simulink model "Microgrid_TLM_server"  (R2025b)
settings: Solver=FixedStepAuto  StartTime=0.0  StopTime=1  FixedStep=5e-7  RelTol=1e-3
InitFcn:
  | clear;
  | setup_two_pc_cosim();
  | clear Server_co Client_co
  | rehash;
  | release_two_pc_tcp_ports();
  | Zc = 45;
  | Vline = 380;%Rated RMS of Line Voltage
  | Vdc = 750;%DC voltage
  | Vac = sqrt(2)*Vline/sqrt(3);%Amplitude of Phase to Neutral Volatge
  | P = 10*10^(3);%Rate Power
  | f=50;%Rated Frequency
  | Wb=2*pi*f;%Rated Angular Frequency
  | fsw1=10e3;  %INV1 switching frequency
  | 
  | %Base Value of PU System
  | Vp=Vac;%Voltage
  | Ip=2/3*P/Vp;%Current
  | Zb = Vp/Ip;%Impedance
  | Lb=Zb/2/pi/f;%Inductance
  | Cb=1/(2*pi*f*Zb);%Capacitance
  | 
  | %Network Parameters
  | R1_pu=0.1/Zb;R1=R1_pu*Zb;
  | R2_pu=0.1/Zb;R2=R2_pu*Zb;
  | R3_pu=0.1/Zb;R3=R3_pu*Zb;
  | R4_pu=0.1/Zb;R4=R4_pu*Zb;
  | L1_pu=2e-3/Lb;L1=L1_pu*Lb;
  | L2_pu=2e-3/Lb;L2=L2_pu*Lb;
  | L3_pu=2e-3/Lb;L3=L3_pu*Lb;
  | L4_pu=2e-3/Lb;L4=L4_pu*Lb;
  | 
  | %Load Parameters
  | Rload1_pu=Vp/Ip/Zb;Rload1=Rload1_pu*Zb;
  | Rload2_pu=Vp/Ip/Zb;Rload2=Rload2_pu*Zb;
  | Rload3_pu=Vp/Ip/Zb;Rload3=Rload3_pu*Zb;
  | 
  | %Virtual Impedance
  | Rv_pu=0.05;
  | Xv_pu=0.2;
  | 
  | Lc=2.5e-3;
StopFcn:
  | %% StopFcn: save TLM server-side results
  | 
  | modelName = bdroot;
  | modelFile = get_param(modelName, 'FileName');
  | 
  | if isempty(modelFile)
  |     modelDir = pwd;
  | else
  |     modelDir = fileparts(modelFile);
  | end
  | 
  | resultDir = fullfile(modelDir, 'result');
  | 
  | if ~exist(resultDir, 'dir')
  |     mkdir(resultDir);
  | end
  | 
  | % Server-side workspace variables
  | variableNames = {
  |     'server_voltage'
  |     'server_current'
  |     'server_PQ'
  | };
  | 
  | serverTLMData = struct();
  | 
  | for k = 1:numel(variableNames)
  | 
  |     originalName = variableNames{k};
  |     saveName = [originalName, '_TLM'];
  | 
  |     if evalin('base', sprintf('exist(''%s'', ''var'')', originalName))
  |         serverTLMData.(saveName) = evalin('base', originalName);
  |     else
  |         warning( ...
  |             'StopFcn:MissingVariable', ...
  |             'Variable "%s" was not found in the base workspace.', ...
  |             originalName);
  |     end
  | end
  | 
  | % Save to result/server_TLM.mat
  | saveFile = fullfile(resultDir, 'server_TLM.mat');
  | save(saveFile, '-struct', 'serverTLMData');
  | 
  | fprintf('TLM server-side results saved to:\n%s\n', saveFile);
undefined symbols (not defined in the file or in its folder): DiscIntNeverNeededParam, Lline1
libraries: spsThreePhaseSeriesRLCBranchLib x14, spsControlledVoltageSourceLib x12, spsThreePhaseVIMeasurementLib x7, spsabctodq0Lib x6, slpidlib x4, spsThreePhaseBreakerLib x4, spsControlledCurrentSourceLib x3, SimplusGT x3, spsPower3phInstantaneousLib x2, spsdq0toabcLib x2, spsThreePhaseTransformerTwoWindingsLib x2, spsDistributedParametersLineLib x1
(part 1 of 2)
settings Model: Creator=L  LastModifiedBy=Zhai Xinjie
settings SolverCC: AlgebraicLoopSolver=TrustRegion
settings DataIOCC: LimitDataPoints=on  SaveFormat=Array  ReturnWorkspaceOutputs=off
settings OptimizationCC: ReuseModelBlockBuffer=off  LifeSpan=inf
settings DebuggingCC: UnderspecifiedInitializationDetection=Classic  MergeDetectMultiDrivingBlocksExec=none  SolverPrmCheckMsg=warning  UnconnectedInputMsg=warning  UnconnectedOutputMsg=warning  UnconnectedLineMsg=warning  StateNameClashWarn=warning  SFUnexpectedBacktrackingDiag=warning  SFNoUnconditionalDefaultTransitionDiag=warning  SFExecutionAtInitializationDiag=none  ArithmeticOperatorsInVariantConditions=warning
settings HardwareCC: ProdBitPerPointer=32.0  ProdBitPerSizeT=32.0  ProdBitPerPtrDiffT=32.0  ProdLargestAtomicFloat=None  ProdIntDivRoundTo=Undefined  ProdEndianess=Unspecified  ProdWordSize=32.0  ProdHWDeviceType=32-bit Generic
settings ModelReferenceCC: EnableRefExpFcnMdlSchedulingChecks=on  PropagateSignalLabelsOutOfModel=off
settings SFSimCC: SimUseLocalCustomCode=off  CustomCodeUndefinedFunction=UseInterfaceOnly
settings RTWCC: RTWUseLocalCustomCode=off  GPUComputeCapability=3.5  DLArmComputeVersion=19.05
settings CodeAppCC: StateflowObjectComments=on
settings GRTTargetCC: TargetLangStandard=C89/C90 (ANSI)
settings ConfigComp: CovMetricSettings=dw  CovSaveCumulativeToWorkspaceVar=on  CovSaveSingleToWorkspaceVar=on  CovExternalEMLEnable=off
settings SimscapeCC: SimscapeNormalizeSystem=off

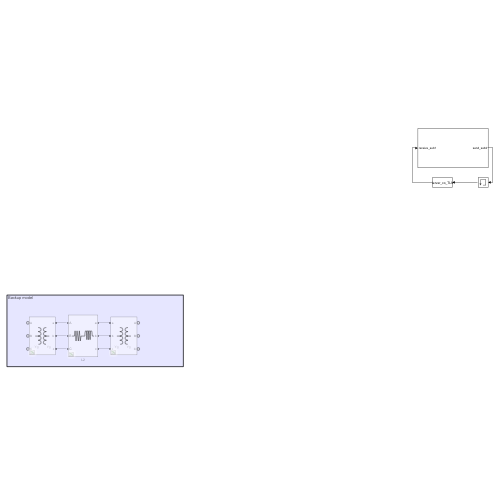
[thumbnail: Simulink's stored preview of the top-level diagram]
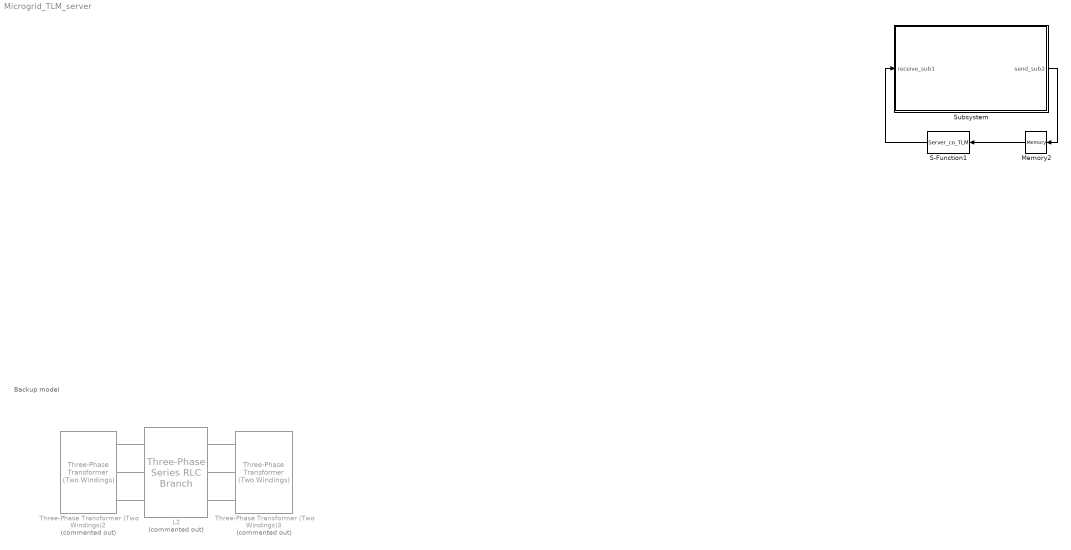
== system Microgrid_TLM_server ==
  note: Backup model
  L2 : spsThreePhaseSeriesRLCBranchLib/Three-Phase Series RLC Branch  Commented=on  LConnTagsString=A|B|C  RConnTagsString=A|B|C  BranchType=RL  Resistance=R2  Inductance=L2  Capacitance=1e-6  Measurements=None
  Memory2 : Memory
  S-Function1 : S-Function  FunctionName=Server_co_TLM  SFunctionDeploymentMode=off  EnableBusSupport=off
  Subsystem : Subsystem
  Three-Phase Transformer (Two Windings)2 : spsThreePhaseTransformerTwoWindingsLib/Three-Phase Transformer (Two Windings)  Commented=on  Winding1Connection=Yg  Winding2Connection=Yg  CoreType=Three single-phase transformers  SetSaturation=off  Hysteresis=off  DataFile='hysteresis'  SetInitialFlux=off  Measurements=None  UNITS=pu  NominalPower=[ 250e6 , 50 ]  Winding1=[ 380e3 , 0.002 , 0.08 ]  Winding2=[ 33e3 , 0.002 , 0.08 ]  Rm=500  Lm=500  L0=0.5  Saturation=[ 0,0 ; 0.0024,1.2 ; 1.0,1.52 ]  InitialFluxes=[ 0.8 , -0.8 , 0.7 ]  BreakLoop=off  DiscreteSolver=Trapezoidal iterative  DataType=off  TransfoNumber=1
  Three-Phase Transformer (Two Windings)3 : spsThreePhaseTransformerTwoWindingsLib/Three-Phase Transformer (Two Windings)  Commented=on  Winding1Connection=Yg  Winding2Connection=Yg  CoreType=Three single-phase transformers  SetSaturation=off  Hysteresis=off  DataFile='hysteresis'  SetInitialFlux=off  Measurements=None  UNITS=pu  NominalPower=[ 250e6 , 50 ]  Winding1=[ 33e3 , 0.002 , 0.08 ]  Winding2=[ 380 , 0.002 , 0.08 ]  Rm=500  Lm=500  L0=0.5  Saturation=[ 0,0 ; 0.0024,1.2 ; 1.0,1.52 ]  InitialFluxes=[ 0.8 , -0.8 , 0.7 ]  BreakLoop=off  DiscreteSolver=Trapezoidal iterative  DataType=off  TransfoNumber=1
  wires:
  Memory2/1 -> S-Function1/1
  Subsystem/1(send_sub2) -> Memory2/1
  S-Function1/1 -> Subsystem/1(receive_sub1)
  connections:
  Three-Phase Transformer (Two Windings)3/RConn1 -- L2/RConn1
  Three-Phase Transformer (Two Windings)3/RConn2 -- L2/RConn2
  Three-Phase Transformer (Two Windings)3/RConn3 -- L2/RConn3
  Three-Phase Transformer (Two Windings)2/RConn1 -- L2/LConn1
  Three-Phase Transformer (Two Windings)2/RConn2 -- L2/LConn2
  Three-Phase Transformer (Two Windings)2/RConn3 -- L2/LConn3

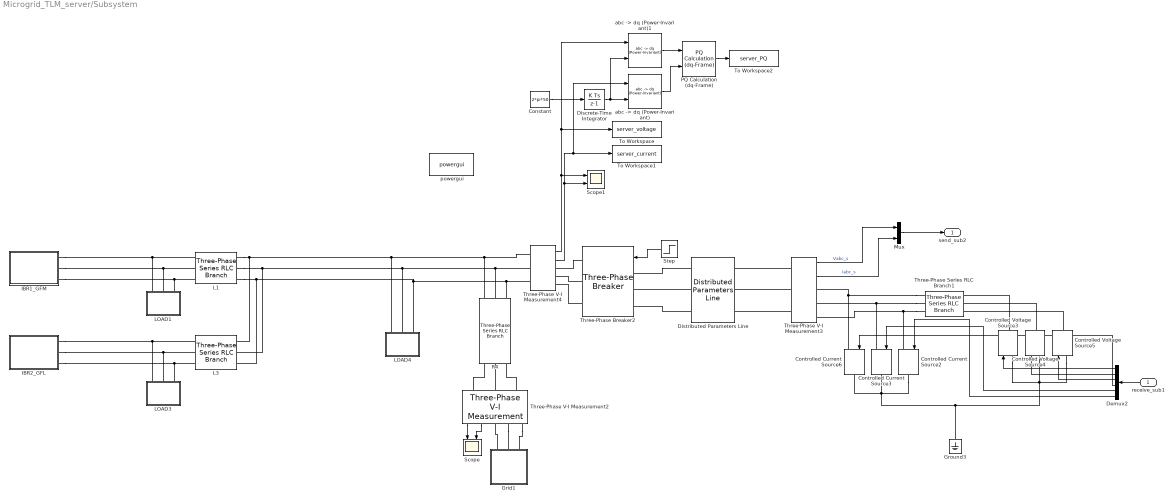
== system Microgrid_TLM_server/Subsystem ==
  receive_sub1 : Inport
  Constant : Constant  Value=2*pi*50
  Controlled Current Source2 : spsControlledCurrentSourceLib/Controlled Current Source  Initialize=on  Source_Type=AC  Amplitude=0  Phase=0  Frequency=0  Measurements=None
  Controlled Current Source3 : spsControlledCurrentSourceLib/Controlled Current Source  Initialize=on  Source_Type=AC  Amplitude=0  Phase=0  Frequency=0  Measurements=None
  Controlled Current Source6 : spsControlledCurrentSourceLib/Controlled Current Source  Initialize=on  Source_Type=AC  Amplitude=0  Phase=0  Frequency=0  Measurements=None
  Controlled Voltage Source3 : spsControlledVoltageSourceLib/Controlled Voltage Source  Initialize=on  Source_Type=AC  Amplitude=0  Phase=0  Frequency=0  Measurements=None
  Controlled Voltage Source4 : spsControlledVoltageSourceLib/Controlled Voltage Source  Initialize=on  Source_Type=AC  Amplitude=0  Phase=0  Frequency=0  Measurements=None
  Controlled Voltage Source5 : spsControlledVoltageSourceLib/Controlled Voltage Source  Initialize=on  Source_Type=AC  Amplitude=0  Phase=0  Frequency=0  Measurements=None
  Demux2 : Demux  Outputs=6
  Discrete-Time Integrator : DiscreteIntegrator  SampleTime=-1  ICPrevOutput=DiscIntNeverNeededParam  ICPrevScaledInput=DiscIntNeverNeededParam
  Distributed Parameters Line : spsDistributedParametersLineLib/Distributed Parameters Line  Phases=3  Length=0.3  Frequency=60  Resistance=[0.075 0.30]  Inductance=[0.30e-3 0.90e-3]  Capacitance=[148e-9 100e-9]  x1=[-3e-06 0 0 0;-2.5e-06 0 0 0;-2e-06 0 0 0;-1.5e-06 0 0 0;-1e-06 0 0 0;-5e-07 0 0 0]  x2=[-3e-06 0 0 0;-2.5e-06 0 0 0;-2e-06 0 0 0;-1.5e-06 0 0 0;-1e-06 0 0 0;-5e-07 0 0 0]  x3=[-3e-06 0 0 0;-2.5e-06 0 0 0;-2e-06 0 0 0;-1.5e-06 0 0 0;-1e-06 0 0 0;-5e-07 0 0 0]  x4=[-3e-06 0 0 0;-2.5e-06 0 0 0;-2e-06 0 0 0;-1.5e-06 0 0 0;-1e-06 0 0 0;-5e-07 0 0 0]  x5=2.84604989415154e-06  V1=ones(3,3)  V2=ones(3,3)  I1=ones(3,3)  I2=ones(3,3)  nHarmo=1  Measurements=None  Decoupling=off  VsMag0=0  VrMag0=0  VsAngle0=0  VrAngle0=0  IsMag0=0  IrMag0=0  IsAngle0=0  IrAngle0=0
      settings: LibrarySourceBlock=sps_lib/Power Grid Elements/Distributed Parameters Line
  Grid1 : Subsystem
  Ground3 : spsGroundLib/Ground  LConnTagsString=a
  IBR1_GFM : Subsystem
  IBR2_GFL : Subsystem
  L1 : spsThreePhaseSeriesRLCBranchLib/Three-Phase Series RLC Branch  LConnTagsString=A|B|C  RConnTagsString=A|B|C  BranchType=RL  Resistance=R1  Inductance=L1  Capacitance=1e-6  Measurements=None
  L3 : spsThreePhaseSeriesRLCBranchLib/Three-Phase Series RLC Branch  LConnTagsString=A|B|C  RConnTagsString=A|B|C  BranchType=RL  Resistance=R3  Inductance=L3  Capacitance=1e-6  Measurements=None
  LOAD1 : Subsystem
  LOAD3 : Subsystem
  LOAD4 : Subsystem
  Mux : Mux  Inputs=2
  PQ Calculation (dq-Frame) : SimplusGT/PQ Calculation (dq-Frame)  SystemSampleTime=-1  VariantActivationTime=update diagram  EmptyChoice=off  PassThrough=off  PassThroughVariantControl=(default)  EmptyChoiceVariantControl=(default)  AllowFlexibleInterface=on  Latency=0  AutoFrameSizeCalculation=off
      settings: SourceProductName=Simplus Grid Tool
  R4 : spsThreePhaseSeriesRLCBranchLib/Three-Phase Series RLC Branch  LConnTagsString=A|B|C  RConnTagsString=A|B|C  BranchType=RL  Resistance=R4  Inductance=L4  Capacitance=1e-6  Measurements=None
  Scope : Scope  NumInputPorts=2
      settings: ActiveDisplayYMinimum=-671.75144212722125  ActiveDisplayYMaximum=671.75144212722125
  Scope1 : Scope  NumInputPorts=2
      settings: ActiveDisplayYMinimum=-701.589020696881  ActiveDisplayYMaximum=701.610214034999  DataLoggingVariableName=ScopeData2
  Step : Step  Time=0.2  SampleTime=0
  Three-Phase Series RLC Branch1 : spsThreePhaseSeriesRLCBranchLib/Three-Phase Series RLC Branch  LConnTagsString=A|B|C  RConnTagsString=A|B|C  BranchType=R  Resistance=Zc  Inductance=1e-3  Capacitance=1e-6  Measurements=None
  Three-Phase V-I Measurement2 : spsThreePhaseVIMeasurementLib/Three-Phase V-I Measurement  VoltageMeasurement=phase-to-phase  SetLabelV=off  LabelV=Vabc1  Vpu=off  VpuLL=off  CurrentMeasurement=yes  SetLabelI=off  LabelI=Iabc3  Ipu=off  Pbase=100e6  Vbase=500e3  OutputType=Complex  PhasorSimulation=off  PSBequivalent=0
  Three-Phase V-I Measurement3 : spsThreePhaseVIMeasurementLib/Three-Phase V-I Measurement  VoltageMeasurement=phase-to-ground  SetLabelV=off  LabelV=Vabc_s  Vpu=off  VpuLL=off  CurrentMeasurement=yes  SetLabelI=off  LabelI=Iabc_s  Ipu=off  Pbase=100e6  Vbase=500e3  OutputType=Complex  PhasorSimulation=off  PSBequivalent=0
  Three-Phase V-I Measurement4 : spsThreePhaseVIMeasurementLib/Three-Phase V-I Measurement  VoltageMeasurement=phase-to-phase  SetLabelV=off  LabelV=Vabc1  Vpu=off  VpuLL=off  CurrentMeasurement=yes  SetLabelI=off  LabelI=Iabc3  Ipu=off  Pbase=100e6  Vbase=500e3  OutputType=Complex  PhasorSimulation=off  PSBequivalent=0
  Three-Phase Breaker2 : spsThreePhaseBreakerLib/Three-Phase Breaker  InitialState=open  SwitchA=on  SwitchB=on  SwitchC=on  SwitchTimes=1.5  External=on  BreakerResistance=0.01  SnubberResistance=1e6  SnubberCapacitance=inf  Measurements=None
  To Workspace : ToWorkspace  VariableName=server_voltage  SaveFormat=Timeseries  SampleTime=-1
  To Workspace1 : ToWorkspace  VariableName=server_current  SaveFormat=Timeseries  SampleTime=-1
  To Workspace2 : ToWorkspace  VariableName=server_PQ  SaveFormat=Timeseries  SampleTime=-1
  "abc -> dq (Power-Invariant)" : SimplusGT/abc -> dq (Power-Invariant)  SystemSampleTime=-1  VariantActivationTime=update diagram  EmptyChoice=off  PassThrough=off  PassThroughVariantControl=(default)  EmptyChoiceVariantControl=(default)  AllowFlexibleInterface=on  Latency=0  AutoFrameSizeCalculation=off
      settings: SourceProductName=Simplus Grid Tool
  "abc -> dq (Power-Invariant)1" : SimplusGT/abc -> dq (Power-Invariant)  SystemSampleTime=-1  VariantActivationTime=update diagram  EmptyChoice=off  PassThrough=off  PassThroughVariantControl=(default)  EmptyChoiceVariantControl=(default)  AllowFlexibleInterface=on  Latency=0  AutoFrameSizeCalculation=off
      settings: SourceProductName=Simplus Grid Tool
  powergui : spspowerguiLib/powergui  Priority=1  SimulationMode=Discrete  SampleTime=5e-7  frequency=60  Iterations=50  frequencyindice=0  Pbase=100e6  ErrMax=1e-4  UnitsV=kV  UnitsW=MW  buscounter=0  FunctionMessages=off  echomessages=off  EnableUseOfTLC=off  CurrentSourceSwitches=off  DisableSnubberDevices=off  DisableRonSwitches=off  DisableVfSwitches=off  DisplayEquations=off  AutomaticDiscreteSolvers=off  SolverType=Tustin/Backward Euler (TBE)  Interpol=off  ExternalGateDelay=off  methode=off  Ts=100  x0status=blocks  SPID=on  SwTol=0  HookPort=off  NonlinearTolerance=1e-4  nMaxIteration=100  ContinueOnMaxIteration=off  RestoreLinks=warning  ResistiveCurrentMeasurement=off  Frange=[0:2:500]  Ylog=off  Xlog=on  ShowGrid=off  save=off  variable=ZData  structure=0  ZoomFFT=off  StartTime=0.0  cycles=1  DisplayStyle=1  fundamental=60  FreqAxis=off  MaxFrequency=1000  frequencyindicesteady=1  RmsSteady=1  display=off
  send_sub2 : Outport
  wires:
  Three-Phase V-I Measurement2/2 -> Scope/2
  Three-Phase V-I Measurement2/1 -> Scope/1
  Step/1 -> Three-Phase Breaker2/1
  Demux2/3 -> Controlled Voltage Source5/1
  Demux2/4 -> Controlled Current Source6/1
  Demux2/2 -> Controlled Voltage Source4/1
  Three-Phase V-I Measurement3/2 -> Mux/2  "Iabc_s"
  Mux/1 -> send_sub2/1
  receive_sub1/1 -> Demux2/1
  Demux2/6 -> Controlled Current Source2/1
  Three-Phase V-I Measurement3/1 -> Mux/1  "Vabc_s"
  Demux2/1 -> Controlled Voltage Source3/1
  Demux2/5 -> Controlled Current Source3/1
  Three-Phase V-I Measurement4/1 -> Scope1/1, "abc -> dq (Power-Invariant)1"/1, To Workspace/1
  Three-Phase V-I Measurement4/2 -> Scope1/2, "abc -> dq (Power-Invariant)"/1, To Workspace1/1
  Discrete-Time Integrator/1 -> "abc -> dq (Power-Invariant)1"/2, "abc -> dq (Power-Invariant)"/2
  Constant/1 -> Discrete-Time Integrator/1
  "abc -> dq (Power-Invariant)1"/1 -> PQ Calculation (dq-Frame)/1
  "abc -> dq (Power-Invariant)"/1 -> PQ Calculation (dq-Frame)/2
  PQ Calculation (dq-Frame)/1 -> To Workspace2/1
  connections:
  IBR1_GFM/RConn2 -- L1/LConn2 -- LOAD1/LConn2
  Three-Phase V-I Measurement3/LConn1 -- Distributed Parameters Line/LConn1
  Grid1/LConn1 -- Three-Phase V-I Measurement2/RConn1
  LOAD4/LConn1 -- Three-Phase V-I Measurement4/LConn1 -- R4/LConn1 -- L1/RConn1 -- L3/RConn1
  Three-Phase V-I Measurement2/LConn3 -- R4/RConn3
  L1/LConn1 -- IBR1_GFM/RConn1 -- LOAD1/LConn1
  L1/RConn2 -- Three-Phase V-I Measurement4/LConn2 -- R4/LConn2 -- LOAD4/LConn2 -- L3/RConn2
  Distributed Parameters Line/RConn3 -- Three-Phase Breaker2/LConn3
  Three-Phase V-I Measurement2/RConn2 -- Grid1/LConn2
  IBR1_GFM/RConn3 -- L1/LConn3 -- LOAD1/LConn3
  L1/RConn3 -- L3/RConn3 -- LOAD4/LConn3 -- Three-Phase V-I Measurement4/LConn3 -- R4/LConn3
  Distributed Parameters Line/RConn1 -- Three-Phase Breaker2/LConn1
  LOAD3/LConn1 -- IBR2_GFL/RConn1 -- L3/LConn1
  IBR2_GFL/RConn2 -- LOAD3/LConn2 -- L3/LConn2
  Three-Phase V-I Measurement3/LConn2 -- Distributed Parameters Line/LConn2
  Distributed Parameters Line/RConn2 -- Three-Phase Breaker2/LConn2
  Three-Phase V-I Measurement3/LConn3 -- Distributed Parameters Line/LConn3
  Three-Phase V-I Measurement2/RConn3 -- Grid1/LConn3
  Three-Phase V-I Measurement2/LConn1 -- R4/RConn1
  IBR2_GFL/RConn3 -- LOAD3/LConn3 -- L3/LConn3
  Three-Phase V-I Measurement2/LConn2 -- R4/RConn2
  Three-Phase Series RLC Branch1/LConn3 -- Controlled Current Source2/LConn1 -- Three-Phase V-I Measurement3/RConn3
  Three-Phase Series RLC Branch1/LConn1 -- Controlled Current Source6/LConn1 -- Three-Phase V-I Measurement3/RConn1
  Three-Phase Series RLC Branch1/LConn2 -- Three-Phase V-I Measurement3/RConn2 -- Controlled Current Source3/LConn1
  Controlled Voltage Source5/LConn1 -- Controlled Current Source6/RConn1 -- Controlled Current Source2/RConn1 -- Controlled Current Source3/RConn1 -- Ground3/LConn1 -- Controlled Voltage Source4/LConn1 -- Controlled Voltage Source3/LConn1
  Controlled Voltage Source5/RConn1 -- Three-Phase Series RLC Branch1/RConn3
  Controlled Voltage Source4/RConn1 -- Three-Phase Series RLC Branch1/RConn2
  Controlled Voltage Source3/RConn1 -- Three-Phase Series RLC Branch1/RConn1
  Three-Phase Breaker2/RConn1 -- Three-Phase V-I Measurement4/RConn1
  Three-Phase Breaker2/RConn2 -- Three-Phase V-I Measurement4/RConn2
  Three-Phase Breaker2/RConn3 -- Three-Phase V-I Measurement4/RConn3

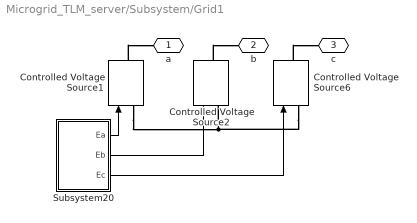
== system Microgrid_TLM_server/Subsystem/Grid1 ==
  Controlled Voltage Source1 : spsControlledVoltageSourceLib/Controlled Voltage Source  Initialize=on  Source_Type=AC  Amplitude=0  Phase=0  Frequency=0  Measurements=None
  Controlled Voltage Source2 : spsControlledVoltageSourceLib/Controlled Voltage Source  Initialize=on  Source_Type=AC  Amplitude=0  Phase=0  Frequency=0  Measurements=None
  Controlled Voltage Source6 : spsControlledVoltageSourceLib/Controlled Voltage Source  Initialize=on  Source_Type=AC  Amplitude=0  Phase=0  Frequency=0  Measurements=None
  Subsystem20 : Subsystem
  a : PMIOPort  Side=Left
  b : PMIOPort  Port=2  Side=Left
  c : PMIOPort  Port=3  Side=Left
  wires:
  Subsystem20/3(Ec) -> Controlled Voltage Source6/1
  Subsystem20/1(Ea) -> Controlled Voltage Source1/1
  Subsystem20/2(Eb) -> Controlled Voltage Source2/1
  connections:
  Controlled Voltage Source1/RConn1 -- a/RConn1
  Controlled Voltage Source6/RConn1 -- c/RConn1
  Controlled Voltage Source6/LConn1 -- Controlled Voltage Source2/LConn1 -- Controlled Voltage Source1/LConn1
  Controlled Voltage Source2/RConn1 -- b/RConn1

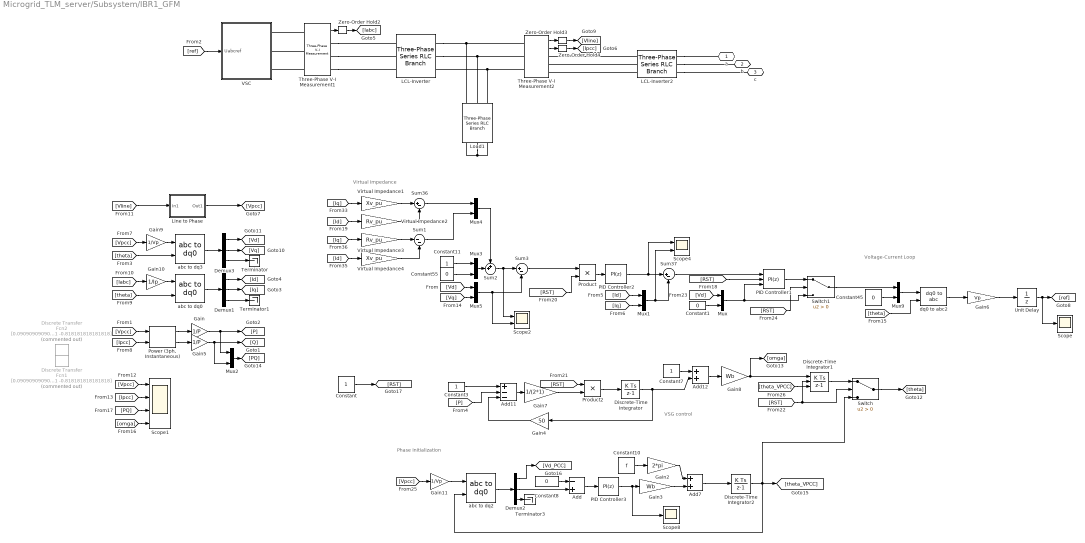
== system Microgrid_TLM_server/Subsystem/IBR1_GFM ==
  note: Voltage-Current Loop
  note: VSG control
  note: Virtual Impedance
  note: Phase Initialization
  Add : Sum  Inputs=-+
  Add11 : Sum  Inputs=+--
  Add12 : Sum
  Add7 : Sum
  Constant : Constant
  Constant{1,8,45,55} (4 alike) : Constant  Value=0
  Constant10 : Constant  Value=f
  Constant11 : Constant  SampleTime=-1
  Constant3 : Constant
  Constant7 : Constant
  Demux1 : Demux  Outputs=3
  Demux2 : Demux  Outputs=3
  Demux3 : Demux  Outputs=3
  Discrete Transfer Fcn1 : DiscreteTransferFcn  Commented=on  Numerator=[0.090909090909091 0.090909090909091]  Denominator=[1 -0.818181818181818]
  Discrete Transfer Fcn2 : DiscreteTransferFcn  Commented=on  Numerator=[0.090909090909091 0.090909090909091]  Denominator=[1 -0.818181818181818]
  Discrete-Time Integrator : DiscreteIntegrator  SampleTime=1/fsw1  ICPrevOutput=DiscIntNeverNeededParam  ICPrevScaledInput=DiscIntNeverNeededParam
  Discrete-Time Integrator1 : DiscreteIntegrator  ExternalReset=rising  InitialConditionSource=external  SampleTime=1/fsw1  ICPrevOutput=DiscIntNeverNeededParam  ICPrevScaledInput=DiscIntNeverNeededParam
  Discrete-Time Integrator2 : DiscreteIntegrator  SampleTime=1/fsw1  ICPrevOutput=DiscIntNeverNeededParam  ICPrevScaledInput=DiscIntNeverNeededParam
  Gain : Gain  Gain=1/P
  Gain10 : Gain  Gain=1/Ip
  Gain11 : Gain  Gain=1/Vp
  Gain2 : Gain  Gain=2*pi
  Gain3 : Gain  Gain=Wb
  Gain4 : Gain  Gain=50
  Gain5 : Gain  Gain=1/P
  Gain6 : Gain  Gain=Vp
  Gain7 : Gain  Gain=1/(2*1)
  Gain8 : Gain  Gain=Wb
  Gain9 : Gain  Gain=1/Vp
  LCL-Inverter : spsThreePhaseSeriesRLCBranchLib/Three-Phase Series RLC Branch  LConnTagsString=A|B|C  RConnTagsString=A|B|C  BranchType=RL  Resistance=0.1  Inductance=2.5e-3  Capacitance=1e-6  Measurements=None
  LCL-Inverter2 : spsThreePhaseSeriesRLCBranchLib/Three-Phase Series RLC Branch  LConnTagsString=A|B|C  RConnTagsString=A|B|C  BranchType=RL  Resistance=0.1  Inductance=0.85e-3  Capacitance=1e-6  Measurements=None
  Line to Phase : Subsystem
  Load1 : spsThreePhaseSeriesRLCBranchLib/Three-Phase Series RLC Branch  LConnTagsString=A|B|C  RConnTagsString=A|B|C  BranchType=RC  Resistance=0.1  Inductance=1e-3  Capacitance=20e-6  Measurements=None
  Mux{,1..5,9} (7 alike) : Mux  Inputs=2
  PID Controller1 : slpidlib/PID Controller  Controller=PI  Form=Parallel  TimeDomain=Discrete-time  UseExternalTs=off  SampleTime=1/fsw1  IntegratorMethod=Forward Euler  FilterMethod=Forward Euler  ControllerParametersSource=internal  P=0.5  I=100  UseKiTs=off  D=0  UseExternalDerivativeSource=off  N=100  UseFilter=on  TunerSelectOption=Transfer Function Based (PID Tuner App)  InitialConditionSource=external  InitialConditionForIntegrator=0  InitialConditionForFilter=0  DifferentiatorICPrevScaledInput=0  ExternalReset=rising  TrackingMode=off  Kt=1  LimitOutput=off  SatLimitsSource=internal  UpperSaturationLimit=inf  LowerSaturationLimit=-inf  LinearizeAsGain=on  AntiWindupMode=none  Kb=1  LimitIntegrator=off  UpperIntegratorSaturationLimit=inf  LowerIntegratorSaturationLimit=-inf  POutMin=[]  POutMax=[]  IOutMin=[]  IOutMax=[]  DOutMin=[]  DOutMax=[]  NOutMin=[]  NOutMax=[]  SumOutMin=[]  SumOutMax=[]  SaturationOutMin=[]  SaturationOutMax=[]  PParamMin=[]  PParamMax=[]  IParamMin=[]  IParamMax=[]  DParamMin=[]  DParamMax=[]  NParamMin=[]  NParamMax=[]  KbParamMin=[]  KbParamMax=[]  KtParamMin=[]  KtParamMax=[]  KbOutMin=[]  KbOutMax=[]  KtOutMin=[]  KtOutMax=[]  IntegratorOutMin=[]  IntegratorOutMax=[]  FilterOutMin=[]  FilterOutMax=[]  SumI1OutMin=[]  SumI1OutMax=[]  SumI2OutMin=[]  SumI2OutMax=[]  SumI3OutMin=[]  SumI3OutMax=[]  SumI4OutMin=[]  SumI4OutMax=[]  SumDOutMin=[]  SumDOutMax=[]  DifferentiatorOutMin=[]  DifferentiatorOutMax=[]  FilterDiffOutCoefMin=[]  FilterDiffOutCoefMax=[]  ReciprocalOutMin=[]  ReciprocalOutMax=[]  SumDenOutMin=[]  SumDenOutMax=[]  SumNumOutMin=[]  SumNumOutMax=[]  DivideOutMin=[]  DivideOutMax=[]  UdiffTsProdOutMin=[]  UdiffTsProdOutMax=[]  NTsProdOutMin=[]  NTsProdOutMax=[]  UintegralTsProdOutMin=[]  UintegralTsProdOutMax=[]  UngainTsProdOutMin=[]  UngainTsProdOutMax=[]  ClampingZeroOutDataTypeStr=Inherit: Inherit via back propagation  ClampingZeroOutMin=[]  ClampingZeroOutMax=[]  FilterDenConstantOutDataTypeStr=Inherit: Inherit via back propagation  FilterDenConstantOutMin=[]  FilterDenConstantOutMax=[]  PCopyOutDataTypeStr=Inherit: Inherit via back propagation  PCopyOutMin=[]  PCopyOutMax=[]  NCopyOutDataTypeStr=Inherit: Inherit via back propagation  NCopyOutMin=[]  NCopyOutMax=[]  IntegratorContinuousStateAttributes=''  IntegratorStateMustResolveToSignalObject=off  IntegratorRTWStateStorageClass=Auto  FilterContinuousStateAttributes=''  FilterStateMustResolveToSignalObject=off  FilterRTWStateStorageClass=Auto  ParallelPVariant=InternalParameters  IdealPVariant=Disabled  IVariant=InternalParameters  DVariant=Disabled  IntegratorVariant=Discrete  SatVariant=Disabled  AWVariant=Passthrough  PCopyVariant=Disabled  TRVariant=Disabled  FdbkBlocksVariant=Forward  IdealPFdbkVariant=Disabled  SatFdbkVariant=Disabled  DerivativeFilterVariant=Disabled  NVariant=Disabled  NCopyVariant=Disabled_SignalSpec  FilterICVariant=Disabled  IntegratorICVariant=ExternalICs  ExternalResetVariant=ExternalReset  TRSumVariant=Passthrough  SumFdbkVariant=Disabled  SumVariant=Sum_PI  TsampFilterVariant=InternalTs  TsampNgainVariant=Passthrough  TsampIntegralVariant=Disabled_SignalSpec  ExternalSaturationOutDataTypeStr=Inherit: Same as second input  DerivativeSourceVariant=Disabled  PreIntVariant=InternalPreInt
  PID Controller2 : slpidlib/PID Controller  Controller=PI  Form=Parallel  TimeDomain=Discrete-time  UseExternalTs=off  SampleTime=1/fsw1  IntegratorMethod=Forward Euler  FilterMethod=Forward Euler  ControllerParametersSource=internal  P=0.2  I=500  UseKiTs=off  D=0  UseExternalDerivativeSource=off  N=100  UseFilter=on  TunerSelectOption=Transfer Function Based (PID Tuner App)  InitialConditionSource=internal  InitialConditionForIntegrator=0  InitialConditionForFilter=0  DifferentiatorICPrevScaledInput=0  ExternalReset=none  TrackingMode=off  Kt=1  LimitOutput=off  SatLimitsSource=internal  UpperSaturationLimit=inf  LowerSaturationLimit=-inf  LinearizeAsGain=on  AntiWindupMode=none  Kb=1  LimitIntegrator=off  UpperIntegratorSaturationLimit=inf  LowerIntegratorSaturationLimit=-inf  POutMin=[]  POutMax=[]  IOutMin=[]  IOutMax=[]  DOutMin=[]  DOutMax=[]  NOutMin=[]  NOutMax=[]  SumOutMin=[]  SumOutMax=[]  SaturationOutMin=[]  SaturationOutMax=[]  PParamMin=[]  PParamMax=[]  IParamMin=[]  IParamMax=[]  DParamMin=[]  DParamMax=[]  NParamMin=[]  NParamMax=[]  KbParamMin=[]  KbParamMax=[]  KtParamMin=[]  KtParamMax=[]  KbOutMin=[]  KbOutMax=[]  KtOutMin=[]  KtOutMax=[]  IntegratorOutMin=[]  IntegratorOutMax=[]  FilterOutMin=[]  FilterOutMax=[]  SumI1OutMin=[]  SumI1OutMax=[]  SumI2OutMin=[]  SumI2OutMax=[]  SumI3OutMin=[]  SumI3OutMax=[]  SumI4OutMin=[]  SumI4OutMax=[]  SumDOutMin=[]  SumDOutMax=[]  DifferentiatorOutMin=[]  DifferentiatorOutMax=[]  FilterDiffOutCoefMin=[]  FilterDiffOutCoefMax=[]  ReciprocalOutMin=[]  ReciprocalOutMax=[]  SumDenOutMin=[]  SumDenOutMax=[]  SumNumOutMin=[]  SumNumOutMax=[]  DivideOutMin=[]  DivideOutMax=[]  UdiffTsProdOutMin=[]  UdiffTsProdOutMax=[]  NTsProdOutMin=[]  NTsProdOutMax=[]  UintegralTsProdOutMin=[]  UintegralTsProdOutMax=[]  UngainTsProdOutMin=[]  UngainTsProdOutMax=[]  ClampingZeroOutDataTypeStr=Inherit: Inherit via back propagation  ClampingZeroOutMin=[]  ClampingZeroOutMax=[]  FilterDenConstantOutDataTypeStr=Inherit: Inherit via back propagation  FilterDenConstantOutMin=[]  FilterDenConstantOutMax=[]  PCopyOutDataTypeStr=Inherit: Inherit via back propagation  PCopyOutMin=[]  PCopyOutMax=[]  NCopyOutDataTypeStr=Inherit: Inherit via back propagation  NCopyOutMin=[]  NCopyOutMax=[]  IntegratorContinuousStateAttributes=''  IntegratorStateMustResolveToSignalObject=off  IntegratorRTWStateStorageClass=Auto  FilterContinuousStateAttributes=''  FilterStateMustResolveToSignalObject=off  FilterRTWStateStorageClass=Auto  ParallelPVariant=InternalParameters  IdealPVariant=Disabled  IVariant=InternalParameters  DVariant=Disabled  IntegratorVariant=Discrete  SatVariant=Disabled  AWVariant=Passthrough  PCopyVariant=Disabled  TRVariant=Disabled  FdbkBlocksVariant=Forward  IdealPFdbkVariant=Disabled  SatFdbkVariant=Disabled  DerivativeFilterVariant=Disabled  NVariant=Disabled  NCopyVariant=Disabled_SignalSpec  FilterICVariant=Disabled  IntegratorICVariant=InternalICs  ExternalResetVariant=Disabled  TRSumVariant=Passthrough  SumFdbkVariant=Disabled  SumVariant=Sum_PI  TsampFilterVariant=InternalTs  TsampNgainVariant=Passthrough  TsampIntegralVariant=Disabled_SignalSpec  ExternalSaturationOutDataTypeStr=Inherit: Same as second input  DerivativeSourceVariant=Disabled  PreIntVariant=InternalPreInt
  PID Controller3 : slpidlib/PID Controller  Controller=PI  Form=Parallel  TimeDomain=Discrete-time  UseExternalTs=off  SampleTime=1/fsw1  IntegratorMethod=Forward Euler  FilterMethod=Forward Euler  ControllerParametersSource=internal  P=2  I=5  UseKiTs=off  D=0  UseExternalDerivativeSource=off  N=100  UseFilter=on  TunerSelectOption=Transfer Function Based (PID Tuner App)  InitialConditionSource=internal  InitialConditionForIntegrator=0  InitialConditionForFilter=0  DifferentiatorICPrevScaledInput=0  ExternalReset=none  TrackingMode=off  Kt=1  LimitOutput=off  SatLimitsSource=internal  UpperSaturationLimit=inf  LowerSaturationLimit=-inf  LinearizeAsGain=on  AntiWindupMode=none  Kb=1  LimitIntegrator=off  UpperIntegratorSaturationLimit=inf  LowerIntegratorSaturationLimit=-inf  POutMin=[]  POutMax=[]  IOutMin=[]  IOutMax=[]  DOutMin=[]  DOutMax=[]  NOutMin=[]  NOutMax=[]  SumOutMin=[]  SumOutMax=[]  SaturationOutMin=[]  SaturationOutMax=[]  PParamMin=[]  PParamMax=[]  IParamMin=[]  IParamMax=[]  DParamMin=[]  DParamMax=[]  NParamMin=[]  NParamMax=[]  KbParamMin=[]  KbParamMax=[]  KtParamMin=[]  KtParamMax=[]  KbOutMin=[]  KbOutMax=[]  KtOutMin=[]  KtOutMax=[]  IntegratorOutMin=[]  IntegratorOutMax=[]  FilterOutMin=[]  FilterOutMax=[]  SumI1OutMin=[]  SumI1OutMax=[]  SumI2OutMin=[]  SumI2OutMax=[]  SumI3OutMin=[]  SumI3OutMax=[]  SumI4OutMin=[]  SumI4OutMax=[]  SumDOutMin=[]  SumDOutMax=[]  DifferentiatorOutMin=[]  DifferentiatorOutMax=[]  FilterDiffOutCoefMin=[]  FilterDiffOutCoefMax=[]  ReciprocalOutMin=[]  ReciprocalOutMax=[]  SumDenOutMin=[]  SumDenOutMax=[]  SumNumOutMin=[]  SumNumOutMax=[]  DivideOutMin=[]  DivideOutMax=[]  UdiffTsProdOutMin=[]  UdiffTsProdOutMax=[]  NTsProdOutMin=[]  NTsProdOutMax=[]  UintegralTsProdOutMin=[]  UintegralTsProdOutMax=[]  UngainTsProdOutMin=[]  UngainTsProdOutMax=[]  ClampingZeroOutDataTypeStr=Inherit: Inherit via back propagation  ClampingZeroOutMin=[]  ClampingZeroOutMax=[]  FilterDenConstantOutDataTypeStr=Inherit: Inherit via back propagation  FilterDenConstantOutMin=[]  FilterDenConstantOutMax=[]  PCopyOutDataTypeStr=Inherit: Inherit via back propagation  PCopyOutMin=[]  PCopyOutMax=[]  NCopyOutDataTypeStr=Inherit: Inherit via back propagation  NCopyOutMin=[]  NCopyOutMax=[]  IntegratorContinuousStateAttributes=''  IntegratorStateMustResolveToSignalObject=off  IntegratorRTWStateStorageClass=Auto  FilterContinuousStateAttributes=''  FilterStateMustResolveToSignalObject=off  FilterRTWStateStorageClass=Auto  ParallelPVariant=InternalParameters  IdealPVariant=Disabled  IVariant=InternalParameters  DVariant=Disabled  IntegratorVariant=Discrete  SatVariant=Disabled  AWVariant=Passthrough  PCopyVariant=Disabled  TRVariant=Disabled  FdbkBlocksVariant=Forward  IdealPFdbkVariant=Disabled  SatFdbkVariant=Disabled  DerivativeFilterVariant=Disabled  NVariant=Disabled  NCopyVariant=Disabled_SignalSpec  FilterICVariant=Disabled  IntegratorICVariant=InternalICs  ExternalResetVariant=Disabled  TRSumVariant=Passthrough  SumFdbkVariant=Disabled  SumVariant=Sum_PI  TsampFilterVariant=InternalTs  TsampNgainVariant=Passthrough  TsampIntegralVariant=Disabled_SignalSpec  ExternalSaturationOutDataTypeStr=Inherit: Same as second input  DerivativeSourceVariant=Disabled  PreIntVariant=InternalPreInt
  "Power (3ph, Instantaneous)" : spsPower3phInstantaneousLib/Power (3ph, Instantaneous)
  Product : Product
  Product2 : Product
  Scope : Scope
      settings: ActiveDisplayYMinimum=-1487.20088  ActiveDisplayYMaximum=1156.37442  DataLoggingVariableName=ScopeData2
  Scope1 : Scope  NumInputPorts=4
      settings: ActiveDisplayYMinimum=-459.19644  ActiveDisplayYMaximum=463.11203  DataLoggingVariableName=ScopeData4
  Scope2 : Scope  NumInputPorts=2
      settings: ActiveDisplayYMinimum=-0.48353  ActiveDisplayYMaximum=1.26771
  Scope4 : Scope  NumInputPorts=2
      settings: ActiveDisplayYMinimum=-1.96338  ActiveDisplayYMaximum=2.79764  DataLoggingVariableName=ScopeData3
  Scope8 : Scope
      settings: ActiveDisplayYMinimum=-0.17841  ActiveDisplayYMaximum=0.07598  DataLoggingVariableName=ScopeData4
  Sum1 : Sum  Inputs=|--
  Sum2 : Sum  Inputs=++|
  Sum3 : Sum  Inputs=|+-
  Sum36 : Sum  Inputs=|+-
  Sum37 : Sum  Inputs=|+-
  Switch : Switch  Criteria=u2 > Threshold  SaturateOnIntegerOverflow=off  InputSameDT=off
  Switch1 : Switch  Criteria=u2 > Threshold  SaturateOnIntegerOverflow=off  InputSameDT=off
  Terminator : Terminator
  Terminator1 : Terminator
  Terminator3 : Terminator
  Three-Phase V-I Measurement1 : spsThreePhaseVIMeasurementLib/Three-Phase V-I Measurement  VoltageMeasurement=no  SetLabelV=off  LabelV=Vabc  Vpu=off  VpuLL=off  CurrentMeasurement=yes  SetLabelI=off  LabelI=Iabc  Ipu=off  Pbase=100e6  Vbase=500e3  OutputType=Complex  PhasorSimulation=off  PSBequivalent=0
  Three-Phase V-I Measurement2 : spsThreePhaseVIMeasurementLib/Three-Phase V-I Measurement  VoltageMeasurement=phase-to-phase  SetLabelV=off  LabelV=Vabc  Vpu=off  VpuLL=off  CurrentMeasurement=yes  SetLabelI=off  LabelI=Iabc  Ipu=off  Pbase=100e6  Vbase=500e3  OutputType=Complex  PhasorSimulation=off  PSBequivalent=0
  Unit Delay : UnitDelay  SampleTime=1/fsw1  HasFrameUpgradeWarning=on
  VSC : Subsystem
  Virtual Impedance1 : Gain  Gain=Xv_pu
  Virtual Impedance2 : Gain  Gain=Rv_pu
  Virtual Impedance3 : Gain  Gain=Rv_pu
  Virtual Impedance4 : Gain  Gain=Xv_pu
  Zero-Order Hold2 : ZeroOrderHold  SampleTime=1/fsw1
  Zero-Order Hold3 : ZeroOrderHold  SampleTime=1/fsw1
  Zero-Order Hold4 : ZeroOrderHold  SampleTime=1/fsw1
  abc to dq0 : spsabctodq0Lib/abc to dq0  Alignment=90 degrees behind phase A axis
  abc to dq2 : spsabctodq0Lib/abc to dq0  Alignment=90 degrees behind phase A axis
  abc to dq3 : spsabctodq0Lib/abc to dq0  Alignment=90 degrees behind phase A axis
  dq0 to abc2 : spsdq0toabcLib/dq0 to abc  Alignment=90 degrees behind phase A axis
  a : PMIOPort  Side=Right
  b : PMIOPort  Port=2  Side=Right
  c : PMIOPort  Port=3  Side=Right
  wires:
  Mux2/1 -> [PQ]
  [omga] -> Scope1/4
  [PQ] -> Scope1/3
  "Power (3ph, Instantaneous)"/1 -> Gain/1
  "Power (3ph, Instantaneous)"/2 -> Gain5/1
  [Ipcc] -> "Power (3ph, Instantaneous)"/2
  [Vpcc] -> "Power (3ph, Instantaneous)"/1
  [ref] -> VSC/1(Uabcref)
  Demux3/2 -> [Vq]
  Constant55/1 -> Mux3/2
  Mux9/1 -> dq0 to abc2/1
  [Vq] -> Mux5/2
  Add12/1 -> Gain8/1
  Constant3/1 -> Add11/1
  Mux3/1 -> Sum2/2
  Discrete-Time Integrator/1 -> Add12/2, Gain4/1
  Gain4/1 -> Add11/3
  [Vpcc] -> Gain9/1
  [Iq] -> Mux1/2
  Demux3/3 -> Terminator/1
  Constant45/1 -> Mux9/2
  Add11/1 -> Gain7/1
  [theta] -> abc to dq3/2
  [P] -> Add11/2
  dq0 to abc2/1 -> Gain6/1
  [Id] -> Mux1/1
  [theta] -> abc to dq0/2
  Unit Delay/1 -> Scope/1, [ref]
  Constant11/1 -> Mux3/1
  [Vd] -> Mux5/1
  PID Controller2/1 -> Scope4/1, Sum37/1
  Mux1/1 -> Scope4/2, Sum37/2
  Demux3/1 -> [Vd]
  Gain6/1 -> Unit Delay/1
  Gain10/1 -> abc to dq0/1
  Mux5/1 -> Sum3/2, Scope2/2
  abc to dq3/1 -> Demux3/1
  Constant7/1 -> Add12/1
  [theta] -> dq0 to abc2/2
  Three-Phase V-I Measurement1/1 -> Zero-Order Hold2/1
  Zero-Order Hold2/1 -> [Iabc]
  Three-Phase V-I Measurement2/2 -> Zero-Order Hold4/1
  Three-Phase V-I Measurement2/1 -> Zero-Order Hold3/1
  Zero-Order Hold3/1 -> [Vline]
  Zero-Order Hold4/1 -> [Ipcc]
  Gain9/1 -> abc to dq3/1
  [Iabc] -> Gain10/1
  abc to dq0/1 -> Demux1/1
  Demux1/1 -> [Id]
  Demux1/3 -> Terminator1/1
  Demux1/2 -> [Iq]
  [Vline] -> Line to Phase/1(In1)
  Line to Phase/1(Out1) -> [Vpcc]
  [Vpcc] -> Scope1/1
  [Ipcc] -> Scope1/2
  Gain/1 -> Mux2/1, [P]
  Gain5/1 -> Mux2/2, [Q]
  [Iq] -> Virtual Impedance3/1
  [Id] -> Virtual Impedance4/1
  [Id] -> Virtual Impedance2/1
  Sum36/1 -> Mux4/1
  [Iq] -> Virtual Impedance1/1
  Virtual Impedance1/1 -> Sum36/1
  Sum1/1 -> Mux4/2
  Virtual Impedance2/1 -> Sum36/2
  Virtual Impedance4/1 -> Sum1/2
  Virtual Impedance3/1 -> Sum1/1
  Mux4/1 -> Sum2/1
  [RST] -> Product/2
  Product/1 -> PID Controller2/1
  [RST] -> PID Controller1/2
  Gain7/1 -> Product2/2
  Product2/1 -> Discrete-Time Integrator/1
  [RST] -> Product2/1
  [RST] -> Switch/2, Discrete-Time Integrator1/2
  PID Controller3/1 -> Scope8/1, Gain3/1
  Constant8/1 -> Add/1
  abc to dq2/1 -> Demux2/1
  Demux2/2 -> Add/2
  Demux2/3 -> Terminator3/1
  [Vpcc] -> Gain11/1
  Constant10/1 -> Gain2/1
  Add/1 -> PID Controller3/1
  Gain2/1 -> Add7/1
  Gain3/1 -> Add7/2
  Discrete-Time Integrator2/1 -> Switch/3, [theta_VPCC], abc to dq2/2
  Gain11/1 -> abc to dq2/1
  Add7/1 -> Discrete-Time Integrator2/1
  Constant1/1 -> Mux/2
  [Vd] -> Mux/1
  Mux/1 -> Switch1/3, PID Controller1/3
  Constant/1 -> [RST]
  Gain8/1 -> Discrete-Time Integrator1/1, [omga]
  [theta_VPCC] -> Discrete-Time Integrator1/3
  Discrete-Time Integrator1/1 -> Switch/1
  Switch/1 -> [theta]
  PID Controller1/1 -> Switch1/1
  Switch1/1 -> Mux9/1
  [RST] -> Switch1/2
  Sum37/1 -> PID Controller1/1
  Sum2/1 -> Scope2/1, Sum3/1
  Sum3/1 -> Product/1
  Demux2/1 -> [Vd_PCC]
  connections:
  LCL-Inverter2/RConn1 -- a/RConn1
  Three-Phase V-I Measurement1/RConn1 -- LCL-Inverter/LConn1
  Load1/LConn2 -- LCL-Inverter/RConn2 -- Three-Phase V-I Measurement2/LConn2
  Load1/LConn3 -- LCL-Inverter/RConn3 -- Three-Phase V-I Measurement2/LConn3
  Load1/LConn1 -- LCL-Inverter/RConn1 -- Three-Phase V-I Measurement2/LConn1
  Three-Phase V-I Measurement1/RConn2 -- LCL-Inverter/LConn2
  Three-Phase V-I Measurement1/RConn3 -- LCL-Inverter/LConn3
  LCL-Inverter2/RConn2 -- b/RConn1
  LCL-Inverter2/LConn1 -- Three-Phase V-I Measurement2/RConn1
  LCL-Inverter2/RConn3 -- c/RConn1
  Load1/RConn3 -- Load1/RConn2 -- Load1/RConn1
  Three-Phase V-I Measurement1/LConn1 -- VSC/RConn1
  Three-Phase V-I Measurement1/LConn2 -- VSC/RConn2
  Three-Phase V-I Measurement1/LConn3 -- VSC/RConn3
  LCL-Inverter2/LConn2 -- Three-Phase V-I Measurement2/RConn2
  LCL-Inverter2/LConn3 -- Three-Phase V-I Measurement2/RConn3

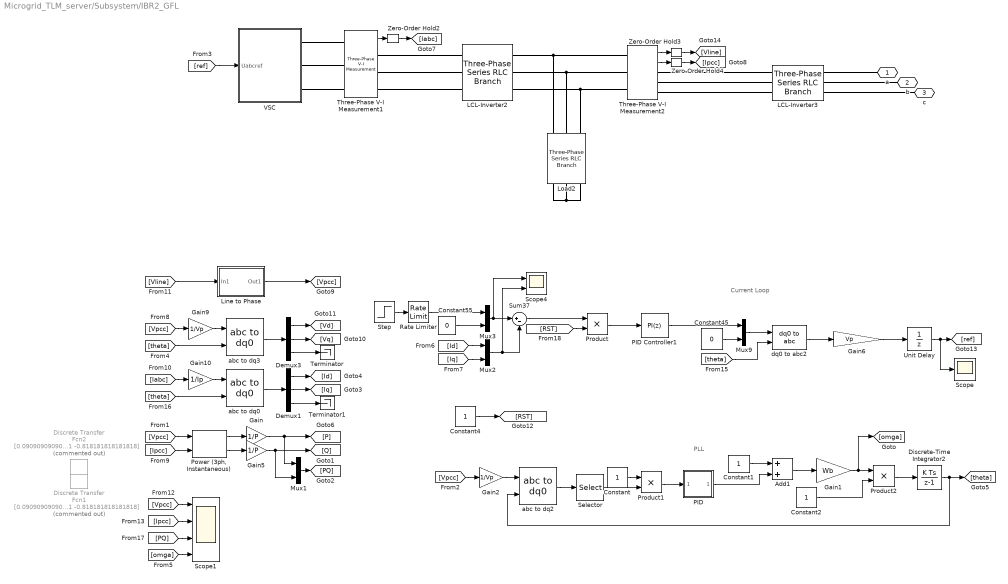
== system Microgrid_TLM_server/Subsystem/IBR2_GFL ==
  note: Current Loop
  note: PLL
  Add1 : Sum
  Constant{,1..2,4} (4 alike) : Constant
  Constant45 : Constant  Value=0
  Constant55 : Constant  Value=0
  Demux1 : Demux  Outputs=3
  Demux3 : Demux  Outputs=3
  Discrete Transfer Fcn1 : DiscreteTransferFcn  Commented=on  Numerator=[0.090909090909091 0.090909090909091]  Denominator=[1 -0.818181818181818]
  Discrete Transfer Fcn2 : DiscreteTransferFcn  Commented=on  Numerator=[0.090909090909091 0.090909090909091]  Denominator=[1 -0.818181818181818]
  Discrete-Time Integrator2 : DiscreteIntegrator  SampleTime=1/fsw1  ICPrevOutput=DiscIntNeverNeededParam  ICPrevScaledInput=DiscIntNeverNeededParam
  Gain : Gain  Gain=1/P
  Gain1 : Gain  Gain=Wb
  Gain10 : Gain  Gain=1/Ip
  Gain2 : Gain  Gain=1/Vp
  Gain5 : Gain  Gain=1/P
  Gain6 : Gain  Gain=Vp
  Gain9 : Gain  Gain=1/Vp
  LCL-Inverter2 : spsThreePhaseSeriesRLCBranchLib/Three-Phase Series RLC Branch  LConnTagsString=A|B|C  RConnTagsString=A|B|C  BranchType=RL  Resistance=0.1  Inductance=2.5e-3  Capacitance=1e-6  Measurements=None
  LCL-Inverter3 : spsThreePhaseSeriesRLCBranchLib/Three-Phase Series RLC Branch  LConnTagsString=A|B|C  RConnTagsString=A|B|C  BranchType=RL  Resistance=0.1  Inductance=0.85e-3  Capacitance=1e-6  Measurements=None
  Line to Phase : Subsystem
  Load2 : spsThreePhaseSeriesRLCBranchLib/Three-Phase Series RLC Branch  LConnTagsString=A|B|C  RConnTagsString=A|B|C  BranchType=RC  Resistance=0.1  Inductance=1e-3  Capacitance=20e-6  Measurements=None
  Mux{1..3,9} (4 alike) : Mux  Inputs=2
  PID : Subsystem
  PID Controller1 : slpidlib/PID Controller  Controller=PI  Form=Parallel  TimeDomain=Discrete-time  UseExternalTs=off  SampleTime=1/fsw1  IntegratorMethod=Forward Euler  FilterMethod=Forward Euler  ControllerParametersSource=internal  P=0.5  I=100  UseKiTs=off  D=0  UseExternalDerivativeSource=off  N=100  UseFilter=on  TunerSelectOption=Transfer Function Based (PID Tuner App)  InitialConditionSource=internal  InitialConditionForIntegrator=[1;0]  InitialConditionForFilter=0  DifferentiatorICPrevScaledInput=0  ExternalReset=none  TrackingMode=off  Kt=1  LimitOutput=off  SatLimitsSource=internal  UpperSaturationLimit=inf  LowerSaturationLimit=-inf  LinearizeAsGain=on  AntiWindupMode=none  Kb=1  LimitIntegrator=off  UpperIntegratorSaturationLimit=inf  LowerIntegratorSaturationLimit=-inf  POutMin=[]  POutMax=[]  IOutMin=[]  IOutMax=[]  DOutMin=[]  DOutMax=[]  NOutMin=[]  NOutMax=[]  SumOutMin=[]  SumOutMax=[]  SaturationOutMin=[]  SaturationOutMax=[]  PParamMin=[]  PParamMax=[]  IParamMin=[]  IParamMax=[]  DParamMin=[]  DParamMax=[]  NParamMin=[]  NParamMax=[]  KbParamMin=[]  KbParamMax=[]  KtParamMin=[]  KtParamMax=[]  KbOutMin=[]  KbOutMax=[]  KtOutMin=[]  KtOutMax=[]  IntegratorOutMin=[]  IntegratorOutMax=[]  FilterOutMin=[]  FilterOutMax=[]  SumI1OutMin=[]  SumI1OutMax=[]  SumI2OutMin=[]  SumI2OutMax=[]  SumI3OutMin=[]  SumI3OutMax=[]  SumI4OutMin=[]  SumI4OutMax=[]  SumDOutMin=[]  SumDOutMax=[]  DifferentiatorOutMin=[]  DifferentiatorOutMax=[]  FilterDiffOutCoefMin=[]  FilterDiffOutCoefMax=[]  ReciprocalOutMin=[]  ReciprocalOutMax=[]  SumDenOutMin=[]  SumDenOutMax=[]  SumNumOutMin=[]  SumNumOutMax=[]  DivideOutMin=[]  DivideOutMax=[]  UdiffTsProdOutMin=[]  UdiffTsProdOutMax=[]  NTsProdOutMin=[]  NTsProdOutMax=[]  UintegralTsProdOutMin=[]  UintegralTsProdOutMax=[]  UngainTsProdOutMin=[]  UngainTsProdOutMax=[]  ClampingZeroOutDataTypeStr=Inherit: Inherit via back propagation  ClampingZeroOutMin=[]  ClampingZeroOutMax=[]  FilterDenConstantOutDataTypeStr=Inherit: Inherit via back propagation  FilterDenConstantOutMin=[]  FilterDenConstantOutMax=[]  PCopyOutDataTypeStr=Inherit: Inherit via back propagation  PCopyOutMin=[]  PCopyOutMax=[]  NCopyOutDataTypeStr=Inherit: Inherit via back propagation  NCopyOutMin=[]  NCopyOutMax=[]  IntegratorContinuousStateAttributes=''  IntegratorStateMustResolveToSignalObject=off  IntegratorRTWStateStorageClass=Auto  FilterContinuousStateAttributes=''  FilterStateMustResolveToSignalObject=off  FilterRTWStateStorageClass=Auto  ParallelPVariant=InternalParameters  IdealPVariant=Disabled  IVariant=InternalParameters  DVariant=Disabled  IntegratorVariant=Discrete  SatVariant=Disabled  AWVariant=Passthrough  PCopyVariant=Disabled  TRVariant=Disabled  FdbkBlocksVariant=Forward  IdealPFdbkVariant=Disabled  SatFdbkVariant=Disabled  DerivativeFilterVariant=Disabled  NVariant=Disabled  NCopyVariant=Disabled_SignalSpec  FilterICVariant=Disabled  IntegratorICVariant=InternalICs  ExternalResetVariant=Disabled  TRSumVariant=Passthrough  SumFdbkVariant=Disabled  SumVariant=Sum_PI  TsampFilterVariant=InternalTs  TsampNgainVariant=Passthrough  TsampIntegralVariant=Disabled_SignalSpec  ExternalSaturationOutDataTypeStr=Inherit: Same as second input  DerivativeSourceVariant=Disabled  PreIntVariant=InternalPreInt
  "Power (3ph, Instantaneous)" : spsPower3phInstantaneousLib/Power (3ph, Instantaneous)
  Product : Product
  Product1 : Product
  Product2 : Product
  Rate Limiter : RateLimiter  RisingSlewLimit=5  FallingSlewLimit=-5  SampleTimeMode=inherited
  Scope : Scope
      settings: ActiveDisplayYMinimum=-423.55092  ActiveDisplayYMaximum=423.50002  DataLoggingVariableName=ScopeData3
  Scope1 : Scope  NumInputPorts=4
      settings: ActiveDisplayYMinimum=-435.11495  ActiveDisplayYMaximum=432.79484  DataLoggingVariableName=ScopeData5
  Scope4 : Scope  NumInputPorts=2
      settings: ActiveDisplayYMinimum=-1.88604  ActiveDisplayYMaximum=1.48102  DataLoggingVariableName=ScopeData8
  Selector : Selector  InputPortWidth=3  IndexOptions=Index vector (dialog)  Indices=[2]  OutputSizes=1
  Step : Step  Time=0  After=0.5  SampleTime=0
  Sum37 : Sum  Inputs=|+-
  Terminator : Terminator
  Terminator1 : Terminator
  Three-Phase V-I Measurement1 : spsThreePhaseVIMeasurementLib/Three-Phase V-I Measurement  VoltageMeasurement=no  SetLabelV=off  LabelV=Vabc  Vpu=off  VpuLL=off  CurrentMeasurement=yes  SetLabelI=off  LabelI=Iabc  Ipu=off  Pbase=100e6  Vbase=500e3  OutputType=Complex  PhasorSimulation=off  PSBequivalent=0
  Three-Phase V-I Measurement2 : spsThreePhaseVIMeasurementLib/Three-Phase V-I Measurement  VoltageMeasurement=phase-to-phase  SetLabelV=off  LabelV=Vabc  Vpu=off  VpuLL=off  CurrentMeasurement=yes  SetLabelI=off  LabelI=Iabc  Ipu=off  Pbase=100e6  Vbase=500e3  OutputType=Complex  PhasorSimulation=off  PSBequivalent=0
  Unit Delay : UnitDelay  SampleTime=1/fsw1  HasFrameUpgradeWarning=on
  VSC : Subsystem
  Zero-Order Hold2 : ZeroOrderHold  SampleTime=1/fsw1
  Zero-Order Hold3 : ZeroOrderHold  SampleTime=1/fsw1
  Zero-Order Hold4 : ZeroOrderHold  SampleTime=1/fsw1
  abc to dq0 : spsabctodq0Lib/abc to dq0  Alignment=90 degrees behind phase A axis
  abc to dq2 : spsabctodq0Lib/abc to dq0  Alignment=90 degrees behind phase A axis
  abc to dq3 : spsabctodq0Lib/abc to dq0  Alignment=90 degrees behind phase A axis
  dq0 to abc2 : spsdq0toabcLib/dq0 to abc  Alignment=90 degrees behind phase A axis
  a : PMIOPort  Side=Right
  b : PMIOPort  Port=2  Side=Right
  c : PMIOPort  Port=3  Side=Right
  wires:
  [Vpcc] -> Gain9/1
  Three-Phase V-I Measurement2/1 -> Zero-Order Hold3/1
  [Vline] -> Line to Phase/1(In1)
  Line to Phase/1(Out1) -> [Vpcc]
  Constant45/1 -> Mux9/2
  dq0 to abc2/1 -> Gain6/1
  Zero-Order Hold2/1 -> [Iabc]
  Three-Phase V-I Measurement1/1 -> Zero-Order Hold2/1
  Demux3/3 -> Terminator/1
  Zero-Order Hold4/1 -> [Ipcc]
  [theta] -> dq0 to abc2/2
  Demux1/2 -> [Iq]
  Gain6/1 -> Unit Delay/1
  abc to dq3/1 -> Demux3/1
  Demux3/1 -> [Vd]
  [Id] -> Mux2/1
  Mux2/1 -> Scope4/2, Sum37/2
  [Iq] -> Mux2/2
  Mux9/1 -> dq0 to abc2/1
  Constant55/1 -> Mux3/2
  [Iabc] -> Gain10/1
  Demux3/2 -> [Vq]
  Demux1/3 -> Terminator1/1
  Gain9/1 -> abc to dq3/1
  Demux1/1 -> [Id]
  Zero-Order Hold3/1 -> [Vline]
  Unit Delay/1 -> Scope/1, [ref]
  [ref] -> VSC/1(Uabcref)
  Three-Phase V-I Measurement2/2 -> Zero-Order Hold4/1
  Gain10/1 -> abc to dq0/1
  [theta] -> abc to dq3/2
  Mux3/1 -> Scope4/1, Sum37/1
  [theta] -> abc to dq0/2
  abc to dq0/1 -> Demux1/1
  Discrete-Time Integrator2/1 -> [theta], abc to dq2/2
  Constant1/1 -> Add1/1
  PID/1(Out1) -> Add1/2
  Add1/1 -> Gain1/1
  abc to dq2/1 -> Selector/1
  PID Controller1/1 -> Mux9/1
  Gain2/1 -> abc to dq2/1
  [Vpcc] -> Gain2/1
  "Power (3ph, Instantaneous)"/1 -> Gain/1
  "Power (3ph, Instantaneous)"/2 -> Gain5/1
  [Ipcc] -> "Power (3ph, Instantaneous)"/2
  [Vpcc] -> "Power (3ph, Instantaneous)"/1
  Gain/1 -> [P], Mux1/1
  [Vpcc] -> Scope1/1
  Gain5/1 -> [Q], Mux1/2
  [PQ] -> Scope1/3
  [Ipcc] -> Scope1/2
  [omga] -> Scope1/4
  Mux1/1 -> [PQ]
  Sum37/1 -> Product/1
  [RST] -> Product/2
  Product/1 -> PID Controller1/1
  Selector/1 -> Product1/2
  Product1/1 -> PID/1(In1)
  Product2/1 -> Discrete-Time Integrator2/1
  Gain1/1 -> [omga], Product2/1
  Constant/1 -> Product1/1
  Constant2/1 -> Product2/2
  Rate Limiter/1 -> Mux3/1
  Step/1 -> Rate Limiter/1
  Constant4/1 -> [RST]
  connections:
  Load2/RConn1 -- Load2/RConn3 -- Load2/RConn2
  LCL-Inverter2/RConn3 -- Load2/LConn3 -- Three-Phase V-I Measurement2/LConn3
  LCL-Inverter2/RConn2 -- Load2/LConn2 -- Three-Phase V-I Measurement2/LConn2
  LCL-Inverter2/RConn1 -- Load2/LConn1 -- Three-Phase V-I Measurement2/LConn1
  LCL-Inverter3/LConn2 -- Three-Phase V-I Measurement2/RConn2
  LCL-Inverter3/LConn3 -- Three-Phase V-I Measurement2/RConn3
  Three-Phase V-I Measurement1/LConn1 -- VSC/RConn1
  LCL-Inverter3/RConn3 -- c/RConn1
  Three-Phase V-I Measurement1/RConn3 -- LCL-Inverter2/LConn3
  Three-Phase V-I Measurement1/RConn2 -- LCL-Inverter2/LConn2
  Three-Phase V-I Measurement1/RConn1 -- LCL-Inverter2/LConn1
  Three-Phase V-I Measurement1/LConn2 -- VSC/RConn2
  LCL-Inverter3/RConn1 -- a/RConn1
  LCL-Inverter3/LConn1 -- Three-Phase V-I Measurement2/RConn1
  Three-Phase V-I Measurement1/LConn3 -- VSC/RConn3
  LCL-Inverter3/RConn2 -- b/RConn1

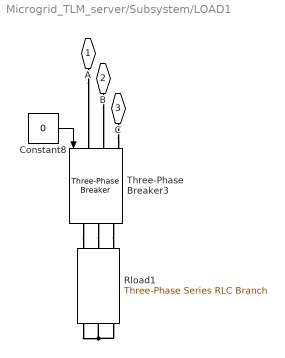
== system Microgrid_TLM_server/Subsystem/LOAD1 ==
  Constant8 : Constant  Value=0
  Rload1 : spsThreePhaseSeriesRLCBranchLib/Three-Phase Series RLC Branch  LConnTagsString=A|B|C  RConnTagsString=A|B|C  BranchType=R  Resistance=Rload1  Inductance=Lline1  Capacitance=1e-6  Measurements=None
  Three-Phase Breaker3 : spsThreePhaseBreakerLib/Three-Phase Breaker  InitialState=open  SwitchA=on  SwitchB=on  SwitchC=on  SwitchTimes=1.5  External=on  BreakerResistance=0.01  SnubberResistance=1e6  SnubberCapacitance=inf  Measurements=None
  A : PMIOPort  Side=Left
  B : PMIOPort  Port=2  Side=Left
  C : PMIOPort  Port=3  Side=Left
  wires:
  Constant8/1 -> Three-Phase Breaker3/1
  connections:
  A/RConn1 -- Three-Phase Breaker3/LConn1
  Three-Phase Breaker3/RConn3 -- Rload1/LConn3
  B/RConn1 -- Three-Phase Breaker3/LConn2
  Rload1/RConn2 -- Rload1/RConn1 -- Rload1/RConn3
  Three-Phase Breaker3/RConn1 -- Rload1/LConn1
  Three-Phase Breaker3/RConn2 -- Rload1/LConn2
  C/RConn1 -- Three-Phase Breaker3/LConn3

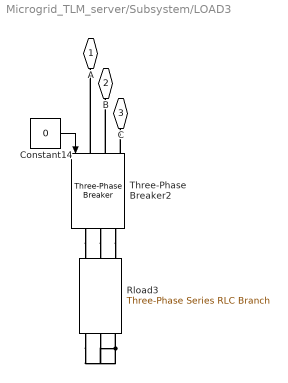
== system Microgrid_TLM_server/Subsystem/LOAD3 ==
  Constant14 : Constant  Value=0
  Rload3 : spsThreePhaseSeriesRLCBranchLib/Three-Phase Series RLC Branch  LConnTagsString=A|B|C  RConnTagsString=A|B|C  BranchType=R  Resistance=Rload3  Inductance=Lline1  Capacitance=1e-6  Measurements=None
  Three-Phase Breaker2 : spsThreePhaseBreakerLib/Three-Phase Breaker  InitialState=open  SwitchA=on  SwitchB=on  SwitchC=on  SwitchTimes=1.5  External=on  BreakerResistance=0.01  SnubberResistance=1e6  SnubberCapacitance=inf  Measurements=None
  A : PMIOPort  Side=Left
  B : PMIOPort  Port=2  Side=Left
  C : PMIOPort  Port=3  Side=Left
  wires:
  Constant14/1 -> Three-Phase Breaker2/1
  connections:
  Three-Phase Breaker2/LConn2 -- B/RConn1
  Three-Phase Breaker2/RConn1 -- Rload3/LConn1
  Three-Phase Breaker2/RConn3 -- Rload3/LConn3
  Rload3/RConn3 -- Rload3/RConn1 -- Rload3/RConn2
  Three-Phase Breaker2/RConn2 -- Rload3/LConn2
  Three-Phase Breaker2/LConn1 -- A/RConn1
  Three-Phase Breaker2/LConn3 -- C/RConn1

== system Microgrid_TLM_server/Subsystem/LOAD4 ==
  Constant1 : Constant
  Rload2 : spsThreePhaseSeriesRLCBranchLib/Three-Phase Series RLC Branch  LConnTagsString=A|B|C  RConnTagsString=A|B|C  BranchType=R  Resistance=Rload2  Inductance=Lline1  Capacitance=1e-6  Measurements=None
  Three-Phase Breaker1 : spsThreePhaseBreakerLib/Three-Phase Breaker  InitialState=open  SwitchA=on  SwitchB=on  SwitchC=on  SwitchTimes=1.5  External=on  BreakerResistance=0.01  SnubberResistance=1e6  SnubberCapacitance=inf  Measurements=None
  A : PMIOPort  Side=Left
  B : PMIOPort  Port=2  Side=Left
  C : PMIOPort  Port=3  Side=Left
  wires:
  Constant1/1 -> Three-Phase Breaker1/1
  connections:
  Three-Phase Breaker1/RConn3 -- Rload2/LConn3
  B/RConn1 -- Three-Phase Breaker1/LConn2
  Three-Phase Breaker1/RConn1 -- Rload2/LConn1
  C/RConn1 -- Three-Phase Breaker1/LConn3
  Rload2/RConn3 -- Rload2/RConn2 -- Rload2/RConn1
  Three-Phase Breaker1/RConn2 -- Rload2/LConn2
  A/RConn1 -- Three-Phase Breaker1/LConn1
